simulink model "M1_motor"  (Simulink 10.2)
settings: Solver=ode4  StartTime=0.0  StopTime=10  FixedStep=T_s  RelTol=1e-3
undefined symbols (not defined in the file): A_v, b_m, b_v, den_filter, J_m, k, L, num_filter, omega_v, R, theta_0, V_bar
settings Model: Creator=ioannis  LastModifiedBy=mfocchi
settings DataIOCC: SaveFormat=Dataset  SignalLoggingSaveFormat=Dataset
settings OptimizationCC: LifeSpan=auto
settings DebuggingCC: UnderspecifiedInitializationDetection=Simplified  MergeDetectMultiDrivingBlocksExec=error  FcnCallInpInsideContextMsg=error  SFUnexpectedBacktrackingDiag=error  SFNoUnconditionalDefaultTransitionDiag=error  SFExecutionAtInitializationDiag=warning
settings HardwareCC: ProdBitPerPointer=64  ProdBitPerSizeT=64  ProdBitPerPtrDiffT=64  ProdLargestAtomicFloat=Float  ProdIntDivRoundTo=Zero  ProdEndianess=LittleEndian  ProdWordSize=64  ProdHWDeviceType=Intel->x86-64 (Windows64)
settings ModelReferenceCC: PropagateSignalLabelsOutOfModel=on
settings SFSimCC: SimUseLocalCustomCode=on
settings RTWCC: RTWUseLocalCustomCode=on
settings CodeAppCC: StateflowObjectComments=off
settings GRTTargetCC: TargetLangStandard=C99 (ISO)  CombineOutputUpdateFcns=on  GRTInterface=off
settings ConfigComp: CovMetricSettings=dwe  CovSaveCumulativeToWorkspaceVar=off  CovSaveSingleToWorkspaceVar=off  CovExternalEMLEnable=on

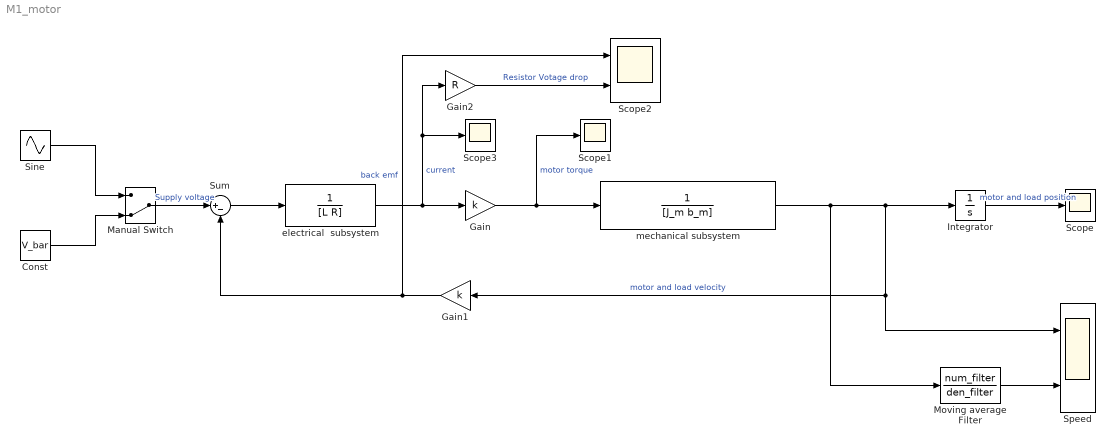
== system M1_motor ==
  "Const " : Constant  Value=V_bar
  Gain : Gain  Gain=k
  Gain1 : Gain  Gain=k
  Gain2 : Gain  Gain=R
  Integrator : Integrator  InitialCondition=theta_0
  Manual Switch : ManualSwitch  CurrentSetting=0
  Moving average Filter : DiscreteFilter  Numerator=num_filter  Denominator=den_filter
  Scope : Scope
  Scope1 : Scope
  Scope2 : Scope  NumInputPorts=2
  Scope3 : Scope
  "Sine " : Sin  Amplitude=A_v  Bias=b_v  Frequency=omega_v  SampleTime=0
  Speed : Scope  NumInputPorts=2
  Sum : Sum  Inputs=|+-
  electrical  subsystem : TransferFcn  Denominator=[L R]
  mechanical subsystem : TransferFcn  Denominator=[J_m b_m]
  wires:
  Gain/1 -> Scope1/1, mechanical subsystem/1  "motor torque"
  mechanical subsystem/1 -> Moving average Filter/1, Speed/1, Gain1/1, Integrator/1  "motor and load velocity"
  Sum/1 -> electrical  subsystem/1
  Gain1/1 -> Scope2/1, Sum/2  "back emf"
  Integrator/1 -> Scope/1  "motor and load position"
  electrical  subsystem/1 -> Gain2/1, Scope3/1, Gain/1  "current"
  "Sine "/1 -> Manual Switch/1
  "Const "/1 -> Manual Switch/2
  Manual Switch/1 -> Sum/1  "Supply voltage"
  Moving average Filter/1 -> Speed/2
  Gain2/1 -> Scope2/2  "Resistor Votage drop"
